simulink model "unicycle_state_error_feedback_linear"  (R2025b)
settings: Solver=ode5  StartTime=0.0  StopTime=40  FixedStep=1e-3  MaxStep=0.01  RelTol=1e-3
libraries: dspsigops x1
settings Model: Creator=Cris  LastModifiedBy=Cris
settings DebuggingCC: UnderspecifiedInitializationDetection=Classic  MergeDetectMultiDrivingBlocksExec=none
settings ModelReferenceCC: PropagateSignalLabelsOutOfModel=off

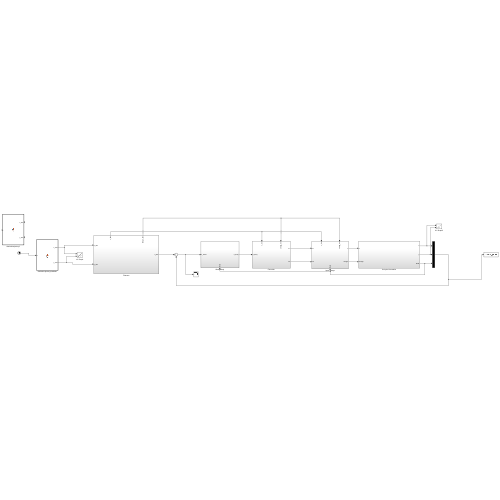
[thumbnail: Simulink's stored preview of the top-level diagram]
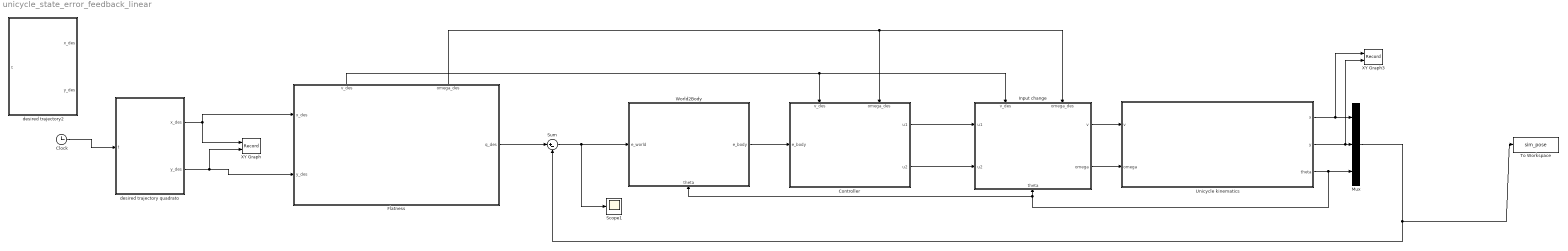
== system unicycle_state_error_feedback_linear ==
  Clock : Clock
  Controller : Subsystem
      settings: PortSchema="{\"entries\":[{\"content\":{\"sides\":[{\"content\":{\"connectorIds\":[\"In1\"]},\"type\":\"ConnectorPlacement.EquallySpacedRectSide\",\"uuid\":\"6a572e67-edde-4e1b-8365-e17ad9f48dde\"},{\"content\":{\"connectorIds\":[\"Out1\",\"Out2\"],\"side\":\"RIGHT\"},\"type\":\"ConnectorPlacement.EquallySpacedRectSide\",\"uuid\":\"eef3ef4a-e0db-4110-95fe-7b093a8263df\"},{\"content\":{\"connectorIds\":[\"In2\",\"In3\"],\"side\":\"TOP\"},\"type\":\"ConnectorPlacement.EquallySpacedRectSide\",\"uuid\":\"36409ed0-e85a-4572-922e-f9880c3e6c77\"}]},\"type\":\"ConnectorPlacement.EquallySpacedConnector\",\"uuid\":\"7cf4f3ea-e25c-438d-a1f8-97a6ff8f9133\"}],\"packageUris\":[\"http://schema.mathworks.com/mf0/Connector/R2020b\"],\"version\":\"1.0\"}"
  Flatness : Subsystem
      settings: PortSchema="{\"entries\":[{\"content\":{\"sides\":[{\"content\":{\"connectorIds\":[\"In1\",\"In2\"]},\"type\":\"ConnectorPlacement.EquallySpacedRectSide\",\"uuid\":\"6c807e7d-3abf-4a72-aeea-144278aa79f3\"},{\"content\":{\"connectorIds\":[\"Out1\"],\"side\":\"RIGHT\"},\"type\":\"ConnectorPlacement.EquallySpacedRectSide\",\"uuid\":\"d7bfc7e3-0ce1-4a6f-8c86-0e8591b05c3c\"},{\"content\":{\"connectorIds\":[\"Out2\",\"Out3\"],\"side\":\"TOP\"},\"type\":\"ConnectorPlacement.EquallySpacedRectSide\",\"uuid\":\"66e20350-45f9-40e8-ade3-59ef62b36a6e\"}]},\"type\":\"ConnectorPlacement.EquallySpacedConnector\",\"uuid\":\"8707f74a-8df1-4d2a-84a5-1332b244f1cc\"}],\"packageUris\":[\"http://schema.mathworks.com/mf0/Connector/R2020b\"],\"version\":\"1.0\"}"
  Input change : Subsystem
      settings: PortSchema="{\"entries\":[{\"content\":{\"sides\":[{\"content\":{\"connectorIds\":[\"In1\",\"In2\"]},\"type\":\"ConnectorPlacement.EquallySpacedRectSide\",\"uuid\":\"644d5157-9aae-4502-a3f2-982c62474d44\"},{\"content\":{\"connectorIds\":[\"Out1\",\"Out2\"],\"side\":\"RIGHT\"},\"type\":\"ConnectorPlacement.EquallySpacedRectSide\",\"uuid\":\"021b21a7-af88-4509-a669-5af41800d21c\"},{\"content\":{\"connectorIds\":[\"In3\",\"In4\"],\"side\":\"TOP\"},\"type\":\"ConnectorPlacement.EquallySpacedRectSide\",\"uuid\":\"7443d77a-8f39-4b3a-bb2e-d99e6d65d58a\"},{\"content\":{\"connectorIds\":[\"In5\"],\"side\":\"BOTTOM\"},\"type\":\"ConnectorPlacement.EquallySpacedRectSide\",\"uuid\":\"7893ab51-5b68-4db3-b1a3-eaaffb015c7e\"}]},\"type\":\"ConnectorPlacement.EquallySpacedConnector\",\"uuid\":\"aa46f843-3616-44ec-bdf9-0b33ba54fabb\"}],\"packageUris\":[\"http://schema.mathworks.com/mf0/Connector/R2020b\"],\"version\":\"1.0\"}"
  Mux : Mux  Inputs=3
  Scope1 : Scope
      settings: ActiveDisplayYMinimum=-1  ActiveDisplayYMaximum=1  DataLoggingVariableName=ScopeData3  DataLoggingSaveFormat=Array
  Sum : Sum  Inputs=|+-
  To Workspace : ToWorkspace  VariableName=sim_pose  SaveFormat=Timeseries  SampleTime=-1
  Unicycle kinematics : Subsystem
  World2Body : Subsystem
      settings: PortSchema="{\"entries\":[{\"content\":{\"sides\":[{\"content\":{\"connectorIds\":[\"In1\"]},\"type\":\"ConnectorPlacement.EquallySpacedRectSide\",\"uuid\":\"d6332ee4-6e37-4568-865c-a04eee2f5a67\"},{\"content\":{\"connectorIds\":[\"Out1\"],\"side\":\"RIGHT\"},\"type\":\"ConnectorPlacement.EquallySpacedRectSide\",\"uuid\":\"8e88a442-f659-4873-b48a-1ad3acef8f2e\"},{\"content\":{\"side\":\"TOP\"},\"type\":\"ConnectorPlacement.EquallySpacedRectSide\",\"uuid\":\"5470688b-b468-4d37-81dc-c9eceb17c0d6\"},{\"content\":{\"connectorIds\":[\"In2\"],\"side\":\"BOTTOM\"},\"type\":\"ConnectorPlacement.EquallySpacedRectSide\",\"uuid\":\"6cdf92e1-737e-401c-b678-b52de2aa14fc\"}]},\"type\":\"ConnectorPlacement.EquallySpacedConnector\",\"uuid\":\"674f477f-0e86-4671-9466-4d2b04f4aa78\"}],\"packageUris\":[\"http://schema.mathworks.com/mf0/Connector/R2020b\"],\"version\":\"1.0\"}"
  XY Graph : Record  NumPorts=2.0  FileSettingsInternal="{\"entries\":[{\"content\":{\"excelSettings\":{\"content\":{},\"type\":\"Streamout.ExcelSettings\"},\"parquetSettings\":{\"content\":{},\"type\":\"Streamout.ParquetSettings\"}},\"type\":\"Streamout.FileSettingStorage\",\"uuid\":\"\"}],\"packageUris\":[\"http:\\/\\/schema.mathworks.com\\/mf0\\/streamout_blocks\\/R2020a\"],\"version\":\"1.0\"}"  FrameSettings=[0, 0]  Layout=[1 1]  SignalsInternal="{\"entries\":[{\"content\":{\"signals\":[{\"content\":{\"blockPath\":[],\"dimensions\":[1],\"domain\":\"\",\"lineColor\":\"#a2142f\",\"plots\":[ 1 ],\"port\":1,\"sid\":[\"\"],\"signalID\":1,\"signalName\":\"desired trajectory quadrato:1\"},\"type\":\"RecordBlkView.Signal\",\"uuid\":\"\"},{\"content\":{\"blockPath\":[],\"dimensions\":[1],\"domain\":\"\",\"lineColor\":\"#139fff\",\"plots\":[ 1 ],\"port\":2,\"sid\":[\"\"],\"signalID\":2,\"signalName\":\"desired trajectory quadrato:2\"},\"type\":\"RecordBlkView.Signal\",\"uuid\":\"\"}]},\"type\":\"RecordBlkView.InputSignals\",\"uuid\":\"\"}],\"packageUris\":[\"http:\\/\\/schema.mathworks.com\\/mf0\\/streamout_blocks\\/R2020a\"],\"version\":\"1.0\"}"  VisualizationBindings="{\"xyplotplugin\":{\"info\":[{\"series\":[{\"bindingParametersList\":[{\"parameter\":\"X-Axis\",\"signalID\":1,\"signalName\":\"desired trajectory quadrato:1\"},{\"parameter\":\"Y-Axis\",\"signalID\":2,\"signalName\":\"desired trajectory quadrato:2\"}],\"seriesID\":0}],\"subplotID\":1}]}}"  CompatibilityTag=XY
  XY Graph3 : Record  NumPorts=2.0  FileSettingsInternal="{\"entries\":[{\"content\":{\"excelSettings\":{\"content\":{},\"type\":\"Streamout.ExcelSettings\"},\"parquetSettings\":{\"content\":{},\"type\":\"Streamout.ParquetSettings\"}},\"type\":\"Streamout.FileSettingStorage\",\"uuid\":\"\"}],\"packageUris\":[\"http:\\/\\/schema.mathworks.com\\/mf0\\/streamout_blocks\\/R2020a\"],\"version\":\"1.0\"}"  FrameSettings=[0, 0]  Layout=[1 1]  SignalsInternal="{\"entries\":[{\"content\":{\"signals\":[{\"content\":{\"blockPath\":[],\"dimensions\":[1],\"domain\":\"\",\"lineColor\":\"#a2142f\",\"plots\":[ 1 ],\"port\":1,\"sid\":[\"\"],\"signalID\":1,\"signalName\":\"Unicycle kinematics:1\"},\"type\":\"RecordBlkView.Signal\",\"uuid\":\"\"},{\"content\":{\"blockPath\":[],\"dimensions\":[1],\"domain\":\"\",\"lineColor\":\"#139fff\",\"plots\":[ 1 ],\"port\":2,\"sid\":[\"\"],\"signalID\":2,\"signalName\":\"Unicycle kinematics:2\"},\"type\":\"RecordBlkView.Signal\",\"uuid\":\"\"}]},\"type\":\"RecordBlkView.InputSignals\",\"uuid\":\"\"}],\"packageUris\":[\"http:\\/\\/schema.mathworks.com\\/mf0\\/streamout_blocks\\/R2020a\"],\"version\":\"1.0\"}"  VisualizationBindings="{\"xyplotplugin\":{\"info\":[{\"series\":[{\"bindingParametersList\":[{\"parameter\":\"X-Axis\",\"signalID\":1,\"signalName\":\"Unicycle kinematics:1\"},{\"parameter\":\"Y-Axis\",\"signalID\":2,\"signalName\":\"Unicycle kinematics:2\"}],\"seriesID\":0}],\"subplotID\":1}]}}"  CompatibilityTag=XY
  desired trajectory quadrato : MATLAB Function  TreatAsAtomicUnit=on
  desired trajectory2 : MATLAB Function  TreatAsAtomicUnit=on
  wires:
  Sum/1 -> World2Body/1(e_world), Scope1/1
  Mux/1 -> Sum/2, To Workspace/1
  desired trajectory quadrato/1(x_des) -> Flatness/1(x_des), XY Graph/1
  desired trajectory quadrato/2(y_des) -> Flatness/2(y_des), XY Graph/2
  Clock/1 -> desired trajectory quadrato/1(t)
  Flatness/1(q_des) -> Sum/1
  World2Body/1(e_body) -> Controller/1(e_body)
  Flatness/2(v_des) -> Input change/3(v_des), Controller/2(v_des)
  Flatness/3(omega_des) -> Input change/4(omega_des), Controller/3(omega_des)
  Controller/1(u1) -> Input change/1(u1)
  Controller/2(u2) -> Input change/2(u2)
  Input change/1(v) -> Unicycle kinematics/1(v)
  Input change/2(omega) -> Unicycle kinematics/2(omega)
  Unicycle kinematics/1(x) -> XY Graph3/1, Mux/1
  Unicycle kinematics/3(theta) -> World2Body/2(theta), Input change/5(theta), Mux/3
  Unicycle kinematics/2(y) -> XY Graph3/2, Mux/2

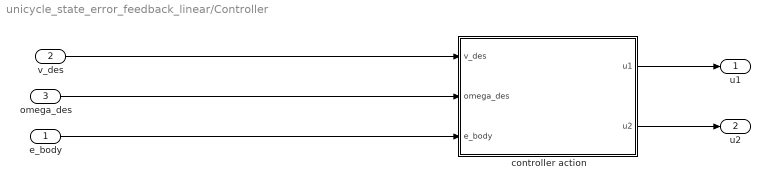
== system unicycle_state_error_feedback_linear/Controller ==
  e_body : Inport
  v_des : Inport  Port=2
  omega_des : Inport  Port=3
  controller action : MATLAB Function  TreatAsAtomicUnit=on
  u1 : Outport
  u2 : Outport  Port=2
  wires:
  v_des/1 -> controller action/1(v_des)
  omega_des/1 -> controller action/2(omega_des)
  e_body/1 -> controller action/3(e_body)
  controller action/1(u1) -> u1/1
  controller action/2(u2) -> u2/1

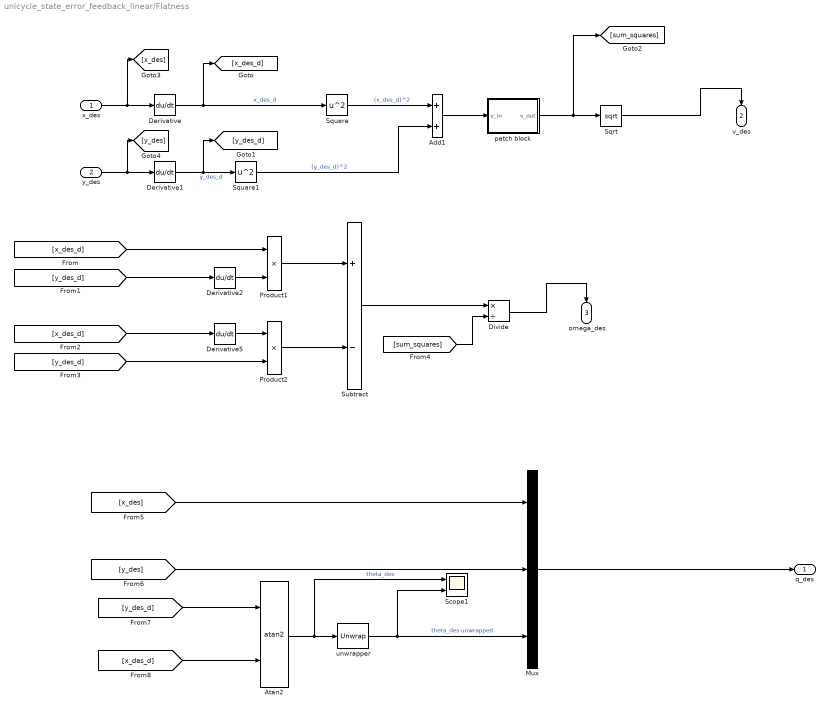
== system unicycle_state_error_feedback_linear/Flatness ==
  x_des : Inport
  y_des : Inport  Port=2
  Add1 : Sum
  Atan2 : Trigonometry  Operator=atan2
  Derivative{,1..2,5} (4 alike) : Derivative
  Divide : Product  Inputs=*/
  Mux : Mux  Inputs=3
  Product1 : Product
  Product2 : Product
  Scope1 : Scope  NumInputPorts=2
      settings: ActiveDisplayYMinimum=-2.3561944901923448  ActiveDisplayYMaximum=5.497787143782138  DataLoggingVariableName=ScopeData2  DataLoggingSaveFormat=Array
  Sqrt : Sqrt
  Square : Math  Operator=square
  Square1 : Math  Operator=square
  Subtract : Sum  Inputs=+-
  patch block : MATLAB Function  TreatAsAtomicUnit=on
  unwrapper : dspsigops/Unwrap  tol=pi  InputProcessing=Columns as channels (frame based)  running=off
  q_des : Outport
  v_des : Outport  Port=2
  omega_des : Outport  Port=3
  wires:
  x_des/1 -> [x_des], Derivative/1
  y_des/1 -> [y_des], Derivative1/1
  Derivative/1 -> [x_des_d], Square/1  "x_des_d"
  Derivative1/1 -> [y_des_d], Square1/1  "y_des_d"
  Square/1 -> Add1/1  "(x_des_d)^2"
  Square1/1 -> Add1/2  "(y_des_d)^2"
  [x_des_d] -> Product1/1
  [y_des_d] -> Derivative2/1
  Derivative2/1 -> Product1/2
  [y_des_d] -> Product2/2
  [x_des_d] -> Derivative5/1
  Derivative5/1 -> Product2/1
  Product1/1 -> Subtract/1
  Product2/1 -> Subtract/2
  Subtract/1 -> Divide/1
  [sum_squares] -> Divide/2
  Divide/1 -> omega_des/1
  Mux/1 -> q_des/1
  Atan2/1 -> unwrapper/1, Scope1/1  "theta_des"
  [x_des_d] -> Atan2/2
  [y_des_d] -> Atan2/1
  Add1/1 -> patch block/1(v_in)
  patch block/1(v_out) -> [sum_squares], Sqrt/1
  Sqrt/1 -> v_des/1
  [x_des] -> Mux/1
  [y_des] -> Mux/2
  unwrapper/1 -> Mux/3, Scope1/2  "theta_des unwrapped"

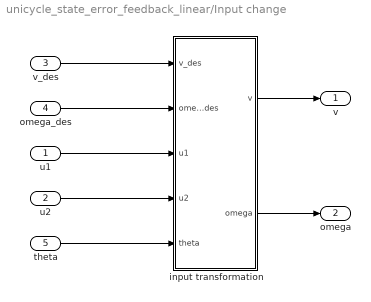
== system unicycle_state_error_feedback_linear/Input change ==
  u1 : Inport
  u2 : Inport  Port=2
  v_des : Inport  Port=3
  omega_des : Inport  Port=4
  theta : Inport  Port=5
  input transformation : MATLAB Function  TreatAsAtomicUnit=on
  v : Outport
  omega : Outport  Port=2
  wires:
  input transformation/2(omega) -> omega/1
  input transformation/1(v) -> v/1
  v_des/1 -> input transformation/1(v_des)
  omega_des/1 -> input transformation/2(omega_des)
  u1/1 -> input transformation/3(u1)
  u2/1 -> input transformation/4(u2)
  theta/1 -> input transformation/5(theta)

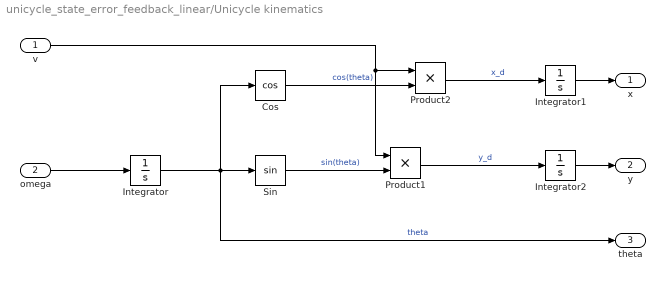
== system unicycle_state_error_feedback_linear/Unicycle kinematics ==
  v : Inport
  omega : Inport  Port=2
  Cos : Trigonometry  Operator=cos
  Integrator : Integrator
  Integrator1 : Integrator
  Integrator2 : Integrator
  Product1 : Product
  Product2 : Product
  Sin : Trigonometry
  x : Outport
  y : Outport  Port=2
  theta : Outport  Port=3
  wires:
  omega/1 -> Integrator/1
  Integrator/1 -> theta/1, Cos/1, Sin/1  "theta"
  Cos/1 -> Product2/2  "cos(theta)"
  Sin/1 -> Product1/2  "sin(theta)"
  v/1 -> Product2/1, Product1/1
  Integrator1/1 -> x/1
  Product2/1 -> Integrator1/1  "x_d"
  Integrator2/1 -> y/1
  Product1/1 -> Integrator2/1  "y_d"

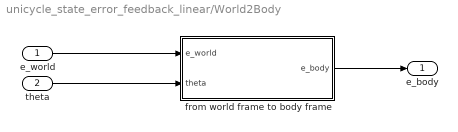
== system unicycle_state_error_feedback_linear/World2Body ==
  e_world : Inport
  theta : Inport  Port=2
  from world frame to body frame : MATLAB Function  TreatAsAtomicUnit=on
  e_body : Outport
  wires:
  e_world/1 -> from world frame to body frame/1(e_world)
  theta/1 -> from world frame to body frame/2(theta)
  from world frame to body frame/1(e_body) -> e_body/1

== matlab function unicycle_state_error_feedback_linear/Controller/controller action ==
  data: v_des input; omega_des input; e_body input; u1 output; u2 output
function [u1, u2] = fcn(v_des, omega_des, e_body)

% TO DO: parametri da modfiicare
d = 1/sqrt(2);
a = 10;



% parametri controllore
k1 = 2*d*a;

% if abs(v_des) < 1e-4
%     if v_des >= 0
%         v_des = 1e-4;
%     else
%         v_des = -1e-4;
%     end
% end

k3 = k1;
k2 = ( a^2-(omega_des)^2 ) / v_des;

u1 = [-k1, 0, 0] * e_body;
u2 = [0, -k2, -k3] * e_body;

== matlab function unicycle_state_error_feedback_linear/World2Body/from world frame to body frame ==
  data: e_world input; e_body output size=3; theta input
function e_body = fcn(e_world, theta)


% Transformation matrix
R = [cos(theta), sin(theta), 0; 
    -sin(theta), cos(theta), 0;
    0, 0, 1];

% get error in body frame
e_body = R*e_world;

== matlab function unicycle_state_error_feedback_linear/Input change/input transformation ==
  data: v_des input; v output size=1; omega_des input; u1 input; u2 input; theta input size=1; omega output
function [v, omega] = fcn(v_des, omega_des, u1, u2, theta)


v = v_des * cos(theta) - u1;
omega = omega_des - u2;

== matlab function unicycle_state_error_feedback_linear/Flatness/patch block ==
  data: v_in input size=1; v_out output size=1
function v_out = fcn(v_in)

if abs(v_in) < 1e-4
    if v_in >= 0
        v_in = 1e-4;
    else
        v_in = -1e-4;
    end
end
v_out = v_in;

== matlab function unicycle_state_error_feedback_linear/desired trajectory quadrato ==
  data: t input; x_des output; y_des output
function [x_des, y_des] = fcn(t)

% % configurable:
% radius = 5;
% omega_des = 0.2;
% 
% % desired trajectory
% x_des = -radius*cos(omega_des*t);
% y_des = -radius*sin(omega_des*t);


% % configurable:
% radius = 10;
% omega_des = 0.5;
% 
% % desired trajectory
% x_des = radius*cos(omega_des*t);
% y_des = radius*sin(omega_des*t);
% 


if t <= 10
    x_des = 10+t;
    y_des = 10;
elseif  t <= 20
    x_des = 20;
    y_des = 0+t;
elseif  t <= 30
    x_des = 40-t;
    y_des = 20;
elseif  t <= 40
    x_des = 10;
    y_des = 50-t;
else
    x_des = 100;
    y_des = 100;
end

== matlab function unicycle_state_error_feedback_linear/desired trajectory2 ==
  data: t input; x_des output; y_des output
function [x_des, y_des] = fcn(t)

% % configurable:
% radius = 5;
% omega_des = 0.2;
% 
% % desired trajectory
% x_des = -radius*cos(omega_des*t);
% y_des = -radius*sin(omega_des*t);


% configurable:
radius = 20;
omega_des = 5;

% desired trajectory
x_des = radius*cos(omega_des*t);
y_des = radius*sin(omega_des*t);



% if t<=10
%     x_des = 10+t;
%     y_des = 10;
% elseif  t<=20
%     x_des = 20;
%     y_des = 10+t;
% elseif  t<=30
%     x_des = 20-t;
%     y_des = 20;
% elseif  t<=40
%     x_des = 10;
%     y_des = 20-t;
% else
%     x_des = 0;
%     y_des = 0;
% end
